simulink model "att2quat"  (R2018a)
settings: Solver=VariableStepAuto  StartTime=0.0  StopTime=10.0  RelTol=1e-3
settings Model: Creator=lamy  LastModifiedBy=lamy

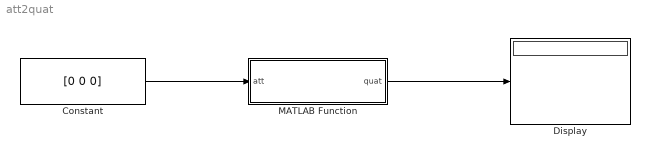
== system att2quat ==
  Constant : Constant  Value=[0 0 0]
  Display : Display
  MATLAB Function : MATLAB Function  TreatAsAtomicUnit=on
  wires:
  Constant/1 -> MATLAB Function/1(att)
  MATLAB Function/1(quat) -> Display/1

== matlab function att2quat/MATLAB Function ==
  data: att input; quat output
function quat = att2quat(att)
quat = [0;0;0;0];
quat(1) = cos(att(1)/2)*cos(att(2)/2)*cos(att(3)/2) + sin(att(1)/2)*sin(att(2)/2)*sin(att(3)/2);
quat(2) = sin(att(1)/2)*cos(att(2)/2)*cos(att(3)/2) - cos(att(1)/2)*sin(att(2)/2)*sin(att(3)/2);
quat(3) = cos(att(1)/2)*sin(att(2)/2)*cos(att(3)/2) + sin(att(1)/2)*cos(att(2)/2)*sin(att(3)/2);
quat(4) = cos(att(1)/2)*cos(att(2)/2)*sin(att(3)/2) - sin(att(1)/2)*sin(att(2)/2)*cos(att(3)/2);
